simulink model "loadcell"  (R2024b)
settings: Solver=FixedStepAuto  StartTime=0.0  StopTime=inf  RelTol=1e-3  EnableMultiTasking=on
libraries: stm32f4xxblockslib x2, simulink x1
settings Model: STM32="{\"AnalogInput\":[{\"ID\":\"untitled:1\"},{\"ID\":\"Poten:1\"},{\"ID\":\"loadcell:74\"}],\"DigitalPortRead\":[{\"ID\":\"untitled:21\"},{\"ID\":\"Poten:21\"},{\"ID\":\"loadcell:91\"}]}"  Creator=rew1m  LastModifiedBy=janej
settings OptimizationCC: DefaultParameterBehavior=Inlined  EnhancedBackFolding=on  PassReuseOutputArgsAs=Individual arguments  ZeroExternalMemoryAtStartup=off  ZeroInternalMemoryAtStartup=off  MaxStackSize=512  OptimizeBlockOrder=speed  DifferentSizesBufferReuse=on  OptimizationCustomize=off  EfficientTunableParamExpr=on
settings DebuggingCC: ParameterTunabilityLossMsg=error
settings HardwareCC: ProdBitPerPointer=32  ProdBitPerSizeT=32  ProdBitPerPtrDiffT=32  ProdLargestAtomicInteger=Long  ProdLargestAtomicFloat=Double  ProdWordSize=32  ProdLongLongMode=on  ProdHWDeviceType=ARM Compatible->ARM Cortex-M
settings SFSimCC: MATLABDynamicMemAlloc=off
settings RTWCC: Description=Embedded Coder  SystemTargetFile=ert.tlc  HardwareBoard=STM32G4xx Based  TemplateMakefile=ert_default_tmf  Toolchain=GNU Tools for ARM Embedded Processors
settings CodeAppCC: ForceParamTrailComments=on  IgnoreCustomStorageClasses=off  OperatorAnnotations=on  SimulinkDataObjDesc=on  SFDataObjDesc=on  InsertBlockDesc=on
settings ERTTargetCC: TargetLangStandard=C99 (ISO)  CodeReplacementLibrary=ARM Cortex-M  ExtModeTransport=3  ExtModeStaticAlloc=on  ExtModeStaticAllocSize=2048  ExtModeMexFile=ext_xcp  ExtModeIntrfLevel=Level2 - Open

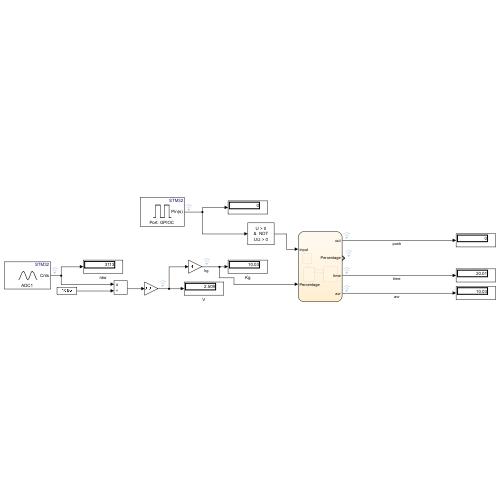
[thumbnail: Simulink's stored preview of the top-level diagram]
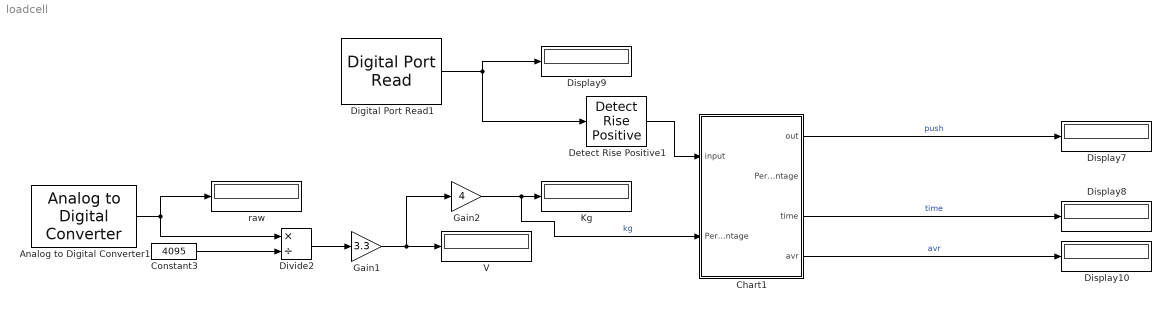
== system loadcell ==
  Analog to Digital Converter1 : stm32f4xxblockslib/Analog to Digital Converter  ADCModule=ADC1  ConversionGroup=Regular  TriggerMode=Trigger and read  NumberOfConversions=1  EnableBufferConv=off  BufferLength=1  OutputStatus=off  SampleTime=-1  EnableSimPort=off  hoistedMaskSrc=ECSoC/ECSimCodegen/Analog to Digital Converter
  Chart1 : Stateflow chart  TreatAsAtomicUnit=on
  Constant3 : Constant  Value=4095
  Detect Rise Positive1 : simulink/Logic and Bit Operations/Detect Rise Positive  vinit=0  OutDataTypeStr=boolean
  Digital Port Read1 : stm32f4xxblockslib/Digital Port Read  PortName=GPIOC  PinNumber=[13]  ReadOperation=on  IOAsArray=on  SampleTime=-1  EnableSimPort=off  hoistedMaskSrc=ECSoC/ECSimCodegen/Digital Port Read
  Display{7..10} (4 alike) : Display
  Divide2 : Product  Inputs=*/
  Gain1 : Gain  Gain=3.3
  Gain2 : Gain  Gain=4
  Kg : Display
  V : Display
  raw : Display
  wires:
  Analog to Digital Converter1/1 -> Divide2/1, raw/1
  Constant3/1 -> Divide2/2
  Divide2/1 -> Gain1/1
  Gain1/1 -> Gain2/1, V/1
  Gain2/1 -> Chart1/2("Percentage "), Kg/1  "kg"
  Chart1/4(avr) -> Display10/1  "avr"
  Chart1/3(time) -> Display8/1  "time"
  Chart1/1(out) -> Display7/1  "push"
  Detect Rise Positive1/1 -> Chart1/1(input)
  Digital Port Read1/1 -> Detect Rise Positive1/1, Display9/1

== stateflow chart loadcell/Chart1 ==
  state Inital
    time = 0;
    out = 0;
    total = 0;
    avr = 0;
    round = 1;
  state HIGHT
    entry:
    out = 1;
    time = 0.01;
    avr = 0;
    during:
    time = time + 0.02
    Percentage = Percentage
    total = total + Percentage
    round = round + 1
  state Low
    entry:
    out = 0;
    avr = total/round
    total = 0;
    round = 0;
  (default) -> Inital
  Inital -> Low
  HIGHT -> Low : [round >= 1000]
  Low -> HIGHT : [input == 1]
  data: out output; Percentage output; input input; time output; Percentage input; avr output; total local; round local
